simulink model "signalbuilder"  (R2018b)
settings: Solver=FixedStepDiscrete  StartTime=0.0  StopTime=10.0  FixedStep=0.02  RelTol=1e-3
undefined symbols (not defined in the file or in its folder): sigbuilder_block
settings Model: Creator=Manivannan  LastModifiedBy=Manivannan

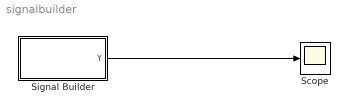
== system signalbuilder ==
  Scope : Scope
  Signal Builder : Subsystem  Tag=STV Subsys  LoadFcn=sigbuilder_block('load');  StartFcn=sigbuilder_block('start');  StopFcn=sigbuilder_block('stop');  ClipboardFcn=sigbuilder_block('clipboard');  mask(Sigbuilder block){tuvar=[0:10]}
      mask help: Simulink:masks:SigbuilderBlock_MD
      mask init:
      | if ~strcmp(get_param(bdroot(gcbh),'SimulationStatus'),'stopped') tuvar = sigbuilder_block('maskInit'); end
      settings: CopyFcn=sigbuilder_block('copy');  DeleteFcn=sigbuilder_block('delete');  ModelCloseFcn=sigbuilder_block('modelClose');  PreSaveFcn=sigbuilder_block('preSave');  PauseFcn=sigbuilder_block('pause');  ContinueFcn=sigbuilder_block('continue');  NameChangeFcn=sigbuilder_block('namechange');  OpenFcn=sigbuilder_block('open',[6 30 1012.5 447.75 ]);  CloseFcn=sigbuilder_block('close');
      mask Display: plot(0, 0, 100, 100,[2, 2, 32, 32, 2], [68, 8, 8, 68, 68],[32, 2], [38, 38], [32, 19, 2],[53, 60, 44], [32, 17, 17, 2],[16, 16, 31, 31]);txt = getActiveGroup(gcbh);text(2, 100, txt,'verticalAlignment', 'top');
  wires:
  Signal Builder/1(Y) -> Scope/1

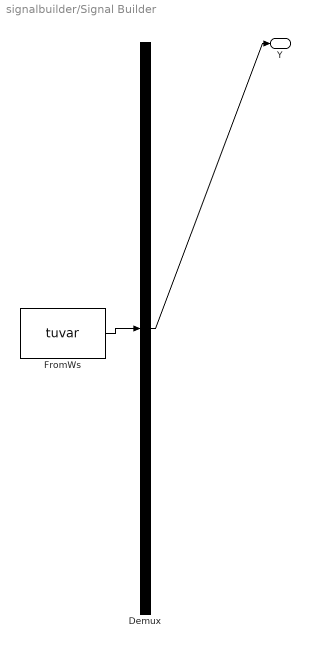
== system signalbuilder/Signal Builder ==
  Demux : Demux  Tag=STV Demux  Outputs=1
  FromWs : FromWorkspace  Tag=STV FromWs  VariableName=tuvar  SampleTime=0
      SigBuilderData=|
      | common.afterFinalStr = 'Extrapolate'
      | common.sampleTime = 0
      | dataSet.timeRange = [0 10.94]
      | dataSet.name = 'Group 1'
      | sbobj.Groups.Name = 'Group 1'
      | sbobj.Groups.Signals.Name = 'Y'
      | sbobj.Groups.Signals.XData = [0 0.36 0.38 0.4 0.42 0.44 0.46 0.48 0.5 0.52 0.54 0.56 ... (531 elements, 1x531)]
      | sbobj.Groups.Signals.YData = [0 -285 15 -70 55 785 992 1007 1003 1002 999 999 1007 1007 1009 1009 993 1007 1008 1008 995 1001 1009 1001 996 1003 1000 1008 1010 1000 1011 996 1008 1000 1005 1007 1006 1005 1008 1005 1004 1008 997 1004 1004 988 935 990 1005 998 946 931 895 824 793 756 706 644 563 468 459 361 316 313 227 198 181 82 25 0 0 1 3 2 0 0 6 0 0 0 0 2 0 0 0 0 0 0 0 0 3 0 6 4 0 0 0 6 0 8 0 0 5 0 0 1 0 3 0 2 1 7 0 0 5 0 9 3 5 7 0 2 0 0 3 0 7 2 0 0 0 7 0 3 7 3 2 2 0 0 0 0 4 7 6 7 2 0 0 0 0 0 1 0 0 0 0 0 3 0 0 4 5 0 5 1 0 7 0 5 0 0 4 2 0 6 4 4 0 1 6 3 0 5 0 1 0 2 4 3 6 7 6 0 0 0 4 5 0 0 0 5 0 0 3 0 0 3 0 3 0 4 0 0 -19.5 0 0 3 0 1 0 4 0 0 4 2 1 0 0 0 6 0 4 0 0 0 6 0 3 0 2 0 4 0 3 0 0 0 0 0 5 5 2 0 0 0 2 4 0 0 4 0 0 0 1 5 0 0 0 0 0 0 0 0 0 0 0 0 4 8 0 0 0 0 5 0 0 4 0 0 9 6 2 0 0 0 5 6 5 0 4 0 0 0 4 0 0 2 0 0 0 0 1 0 1 0 5 2 0 0 0 0 3 1 7 1 0 0 4 0 6 3 0 5 0 0 6 0 4 0 7 0 4 7 0 9 2 3 2 0 0 0 10 3 0 0 29 26 0 50 60 101 83 32 36 69 113 114 61 41 80 118 145 83 66 97 101 119 66 50 63 112 93 5 5 6 80 81 12 48 67 120 136 76 87 97 127 129 108 107 122 158 200 162 138 145 210 235 205 223 249 279 274 280 299 345 376 419 337 361 413 454 500 441 475 490 551 568 517 587 574 626 646 582 669 658 714 764 677 720 753 806 878 818 797 711 716 761 717 637 1 4 0 1 0 0 0 0 0 0 2 0 1 0 8 1 8 0 0 0 4 0 0 2 0 0 0 2 0 2 0 2 5 0 0 3 0 2 0 0 2 0 0 2 0 0 1 3 2 0 4 5 0 5 0 5 5 4 4 0 6 0 0 5 0 0 0 0 8 0 0 4 0 1 0 0 0 0 0 1 5]
      | sbobj.Groups.TimeRange = [0 10.94]
  Y : Outport  Tag=STV Outport
  wires:
  FromWs/1 -> Demux/1
  Demux/1 -> Y/1
